simulink model "FFT_64_Point"  (R2022a)
settings: Solver=VariableStepAuto  StartTime=0.0  StopTime=5000  RelTol=1e-3
undefined symbols (not defined in the file): xc7s100fgga676
libraries: hdlBasic x10, commrandsrc3 x1, vmcUtilities x1
settings Model: Creator=Sandesh  LastModifiedBy=Sandesh

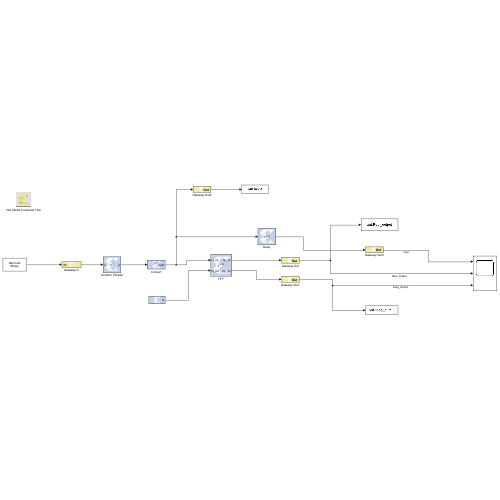
[thumbnail: Simulink's stored preview of the top-level diagram]
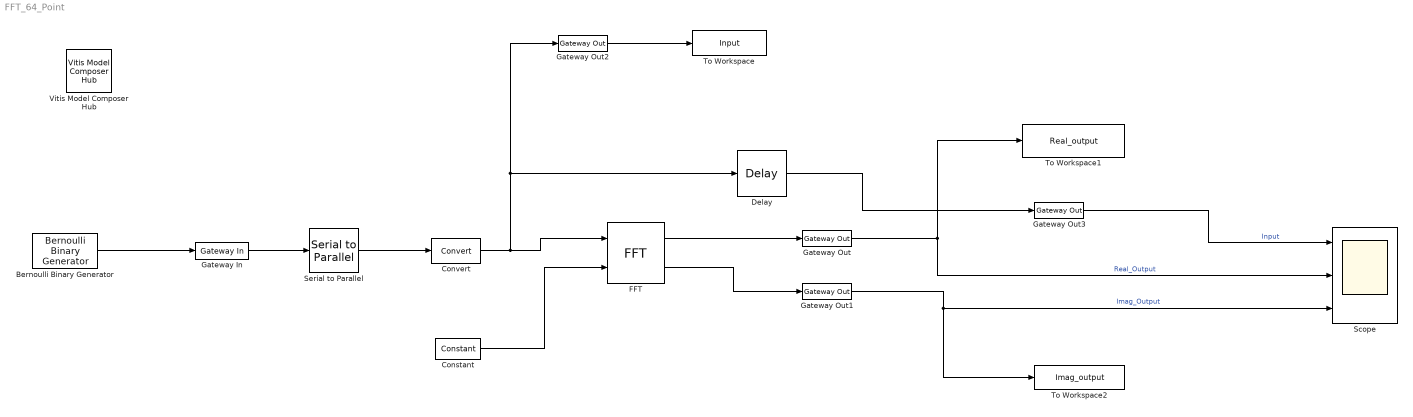
== system FFT_64_Point ==
  Bernoulli Binary Generator : commrandsrc3/Bernoulli Binary Generator  ProbabilityOfZero=0.5  SeedSource=Auto  Seed=0  SampleTime=1  SamplesPerFrame=1  OutputDataType=double  SimulateUsing=Interpreted execution
  Constant : hdlBasic/Constant  const=0  gui_display_data_type=Fixed-point  arith_type=Signed (2's comp)  n_bits=16  bin_pt=0  preci_type=Single  exp_width=8  frac_width=24  explicit_period=off  period=1  XmcBlockStatus=1  maskContainerNames=tabcontainer1  block_type=constant  block_config=sysgen:Constant_config
  Convert : hdlBasic/Convert  gui_display_data_type=Fixed-point  arith_type=Signed (2's comp)  n_bits=16  bin_pt=0  float_type=Single  exp_bits=8  fraction_bits=24  quantization=Truncate  overflow=Wrap  en=off  latency=1  pipeline=off  XmcBlockStatus=1  maskContainerNames=group2  block_type=convert  block_config=sysgen:Convert_config  block_width=595  block_height=885
  Delay : hdlBasic/Delay  rst=off  en=off  latency=214  reg_retiming=off  XmcBlockStatus=1  maskContainerNames=group1  block_type=delay  block_config=sysgen:Delay_config
  FFT : hdlBasic/FFT  transform_length=64  scale_result_by_fft_length=off  bit_reversed_order=on  optimizegoal=Performance  start_frame=off  simulation_type=fast_sim  simulation_model=sysgen:ForwardFFT_Macro  latency=1  XmcBlockStatus=1  maskContainerNames=group1  block_type=xfft_forward  block_config=sysgen:FFTMacro_config
  Gateway In : hdlBasic/Gateway In  gui_display_data_type=Fixed-point  arith_type=Unsigned  n_bits=1  bin_pt=0  preci_type=Single  exp_width=8  frac_width=24  rows=1  columns=1  quantization="Round  (unbiased: +/- Inf)"  overflow=Saturate  period=1  UseAsADC=off  ADCChannel='1'  interface=None  automatic_assignment=on  address_offset=hex2dec('00')  intf_name=''  intf_description=''  default_value=0  timing_constraint=None  locs_specified=off  LOCs={}  io_standard={}  inherit_from_input=off  hdl_port=on  XmcBlockStatus=1  maskContainerNames=group4  block_type=gatewayin  block_config=sysgen:gateway_in_config  block_width_w=590  block_height_w=620  block_width=640  block_height=850
  Gateway Out{,1..3} (4 alike) : hdlBasic/Gateway Out  inherit_from_input=off  hdl_port=on  rows=1  columns=1  UseAsDAC=off  DACChannel='1'  interface=None  automatic_assignment=on  address_offset=hex2dec('00')  intf_name=''  intf_description=''  timing_constraint=None  locs_specified=off  LOCs={}  io_standard={}  XmcBlockStatus=1  maskContainerNames=group4  block_type=gatewayout  block_config=sysgen:gateway_out_config  block_width_w=590  block_height_w=620  block_width=620  block_height=750
  Scope : Scope  NumInputPorts=3
  Serial to Parallel : hdlBasic/Serial to Parallel  input_order=Least Significant Word First  arith_type=Unsigned  output_bits=4  bin_pt=0  rst=off  en=off  latency=1  input_bits=[]  XmcBlockStatus=1  maskContainerNames=group3  block_type=s2p  block_config=sysgen:S2P_config
  To Workspace : ToWorkspace  VariableName=Input  SaveFormat=Timeseries  SampleTime=-1
  To Workspace1 : ToWorkspace  VariableName=Real_output  SaveFormat=Timeseries  SampleTime=-1
  To Workspace2 : ToWorkspace  VariableName=Imag_output  SaveFormat=Timeseries  SampleTime=-1
  Vitis Model Composer Hub : vmcUtilities/Vitis Model Composer Hub  Tag=genX  CodeGeneration=off  TargetDirectory=./code  ExportType=AI Engines  IpVendor=xilinx.com  IpLibrary=hls  IpVersion=1.0  IpHWLanguage=Verilog  AieCompilerOptions={}  CreateTestbench=off  TestbenchStackSize=10  RunAieSim=off  AieSimTimeout=50000  RunAieSimProfiling=off  LaunchVitisAnalyzer=off  PlotOutput=off  RunX86Sim=off  X86SimTimeout=10  GenHwImage=off  PlatformType=Not Specified  HwSystemType=Baremetal  HwValidationTarget=hw  ProjDevice=Spartan-7 SP701 Evaluation Platform (xc7s100fgga676-2)  ProjDevicePart=xc7s100fgga676-2  SamplePeriod=-1  ClockFrequency=200  DataPathParallelism=1  xilinxfamily=spartan7  part=xc7s100  speed=-2  package=fgga676  directory=./netlist  testbench=off  incr_netlist=off  synthesis_tool=Vivado  clock_wrapper=Clock Enables  dbl_ovrd=According to Block Masks  dcm_input_clock_period=10  sysclk_period=10  simulink_period=1  eval_field=0
  wires:
  Bernoulli Binary Generator/1 -> Gateway In/1
  Gateway In/1 -> Serial to Parallel/1
  Convert/1 -> Gateway Out2/1, Delay/1, FFT/1
  Constant/1 -> FFT/2
  FFT/1 -> Gateway Out/1
  FFT/2 -> Gateway Out1/1
  Gateway Out/1 -> Scope/2, To Workspace1/1  "Real_Output"
  Gateway Out1/1 -> To Workspace2/1, Scope/3  "Imag_Output"
  Serial to Parallel/1 -> Convert/1
  Gateway Out2/1 -> To Workspace/1
  Gateway Out3/1 -> Scope/1  "Input"
  Delay/1 -> Gateway Out3/1
